simulink model "pwmCnvCh6"  (R2014a)
settings: configuration reference "globalConfig" (kept outside this file)
undefined symbols (not defined in the file): gcbh, rmidispblock, Ts
settings Model: RequirementInfo={'other' 'throttleReqsCh6.doc' '@pwm_1' 'true' 'Duty cycle must be proportional to controller output, when in a valid range.' '' ; 'other' 'throttleReqsCh6.doc' '@pwm_2' 'true' 'PWM torque should act in positive sense when controller output is positive or zero.' '' ; 'other' 'throttleReqsCh6.doc' '@pwm_3' 'true' 'PWM torque should act in negative sense when controller output is negative.' '' ; 'other' 'throttleReqsCh6.doc' '@pwm_4' 'true' 'Duty cycle must be in range from 0 to 1.' '' } %GIDa_9cd6bfe3_9e51_41b9_91c5_89e7b64823b3  Creator=jrivitus  LastModifiedBy=scastro

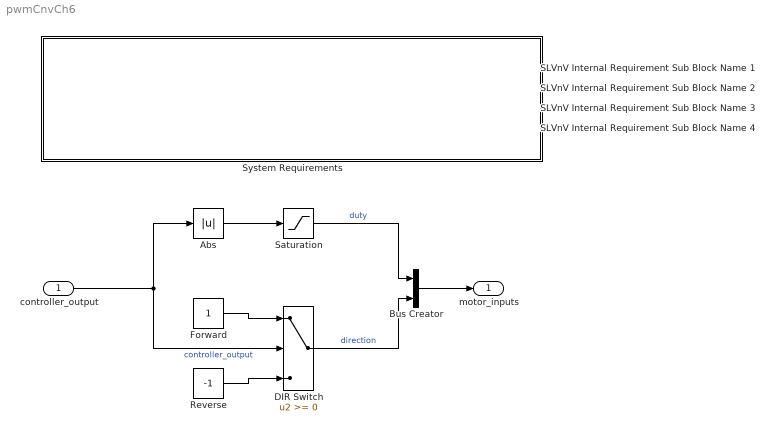
== system pwmCnvCh6 ==
  controller_output : Inport  OutDataTypeStr=double  PortDimensions=1  SampleTime=Ts
  Abs : Abs
  Bus Creator : BusCreator  Inputs=2  OutDataTypeStr=Bus: motor_inputs_bus
  DIR Switch : Switch
      settings: AttributesFormatString=Criteria: %<Criteria>\nThreshold: %<Threshold>
  Forward : Constant  OutDataTypeStr=double
  Reverse : Constant  Value=-1  OutDataTypeStr=double
  SLVnV Internal Requirement Sub Block Name 1 : Subsystem  mask(System Requirement Item){label=0, index=1}
      mask init:
      | label = rmidispblock('label',index);
      settings: CopyFcn=rmidispblock('copyReq',gcbh)  DeleteFcn=rmidispblock('deleteReq',gcbh);  OpenFcn=rmidispblock('openReq',gcbh)  MoveFcn=rmidispblock('move',gcbh);
      mask Display: text(0,0,label,'horizontalAlignment','left','verticalAlignment','bottom')
  SLVnV Internal Requirement Sub Block Name 2 : Subsystem  mask(System Requirement Item){label=0, index=2}
      mask init:
      | label = rmidispblock('label',index);
      settings: CopyFcn=rmidispblock('copyReq',gcbh)  DeleteFcn=rmidispblock('deleteReq',gcbh);  OpenFcn=rmidispblock('openReq',gcbh)  MoveFcn=rmidispblock('move',gcbh);
      mask Display: text(0,0,label,'horizontalAlignment','left','verticalAlignment','bottom')
  SLVnV Internal Requirement Sub Block Name 3 : Subsystem  mask(System Requirement Item){label=0, index=3}
      mask init:
      | label = rmidispblock('label',index);
      settings: CopyFcn=rmidispblock('copyReq',gcbh)  DeleteFcn=rmidispblock('deleteReq',gcbh);  OpenFcn=rmidispblock('openReq',gcbh)  MoveFcn=rmidispblock('move',gcbh);
      mask Display: text(0,0,label,'horizontalAlignment','left','verticalAlignment','bottom')
  SLVnV Internal Requirement Sub Block Name 4 : Subsystem  mask(System Requirement Item){label=0, index=4}
      mask init:
      | label = rmidispblock('label',index);
      settings: CopyFcn=rmidispblock('copyReq',gcbh)  DeleteFcn=rmidispblock('deleteReq',gcbh);  OpenFcn=rmidispblock('openReq',gcbh)  MoveFcn=rmidispblock('move',gcbh);
      mask Display: text(0,0,label,'horizontalAlignment','left','verticalAlignment','bottom')
  Saturation : Saturate  UpperLimit=1  LowerLimit=0
      settings: AttributesFormatString=%<LowerLimit> < duty < %<UpperLimit>
  System Requirements : Subsystem  LoadFcn=rmidispblock('load',gcbh)  mask(System Requirements){id=SystemReq, title=System Requirements}
      mask prompts: title "Block Title"
      mask help: Lists the requirements for the current model.
      mask init:
      | id = 'SystemReq';
      | [w,h] = rmidispblock('display',gcbh);
      settings: CopyFcn=rmidispblock('create',gcbh)  DeleteFcn=rmidispblock('delete',gcbh)  ModelCloseFcn=rmidispblock('close',gcbh)  PreSaveFcn=rmidispblock('close',gcbh)  PostSaveFcn=rmidispblock('open',gcbh)  OpenFcn=rmidispblock('open',gcbh)  MoveFcn=rmidispblock('move',gcbh)
      mask Help: helpview(fullfile(docroot,'toolbox','slvnv','slvnv.map'),'systemrequirements')
      mask Display: text(497/2,121-4,rmidispblock('title',gcbh),'horizontalAlignment','center','verticalAlignment','top')
  motor_inputs : Outport  OutDataTypeStr=Bus: motor_inputs_bus  SampleTime=Ts
  wires:
  Bus Creator/1 -> motor_inputs/1
  Abs/1 -> Saturation/1
  Saturation/1 -> Bus Creator/1  "duty"
  DIR Switch/1 -> Bus Creator/2  "direction"
  Reverse/1 -> DIR Switch/3
  Forward/1 -> DIR Switch/1
  controller_output/1 -> DIR Switch/2, Abs/1  "controller_output"

== system pwmCnvCh6/SLVnV Internal Requirement Sub Block Name 1 ==

== system pwmCnvCh6/SLVnV Internal Requirement Sub Block Name 2 ==

== system pwmCnvCh6/SLVnV Internal Requirement Sub Block Name 3 ==

== system pwmCnvCh6/SLVnV Internal Requirement Sub Block Name 4 ==

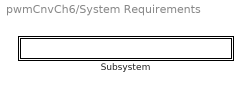
== system pwmCnvCh6/System Requirements ==
  Subsystem : Subsystem  mask{label=0, index=1}
      mask init:
      | label = rmidispblock('label',index);
      settings: OpenFcn=rmidispblock('openReq',gcbh);
      mask Display: text(0,0,label,'horizontalAlignment','left','verticalAlignment','bottom')

== system pwmCnvCh6/System Requirements/Subsystem ==
